simulink model "comfort"  (R2013b)
settings: Solver=ode45  StartTime=0.0  StopTime=0  RelTol=1e-3
undefined symbols (not defined in the file): CarnotCallbacks_PMV_PPD
settings Model: Creator=awohlfei  LastModifiedBy=drhf
settings DebuggingCC: SolverPrmCheckMsg=none  StateNameClashWarn=warning

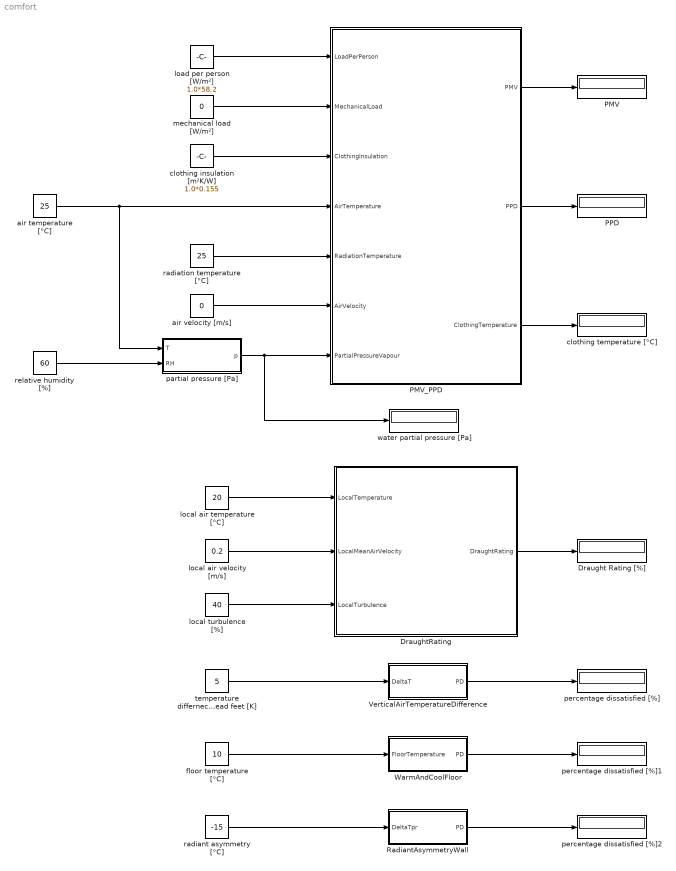
== system comfort ==
  Draught Rating [%] : Display
  DraughtRating : Subsystem  mask(Drauting Rate){}
      mask help: The block calculates the draut rate according to ISO 7730.
  PMV : Display
  PMV_PPD : Subsystem  LoadFcn=CarnotCallbacks_PMV_PPD('LoadFcn', gcb);  mask(PMV_PPD){DEBUGLEVEL=WARNINGLEVEL, MAXTOTALWARNINGS=inf, MAXCONSECUTIVEWARNINGS=inf, WRITETOFILE=0, FILENAME='messages.txt'}
      mask prompts: DEBUGLEVEL "Debug level"; MAXTOTALWARNINGS "maximum number of total warning"; MAXCONSECUTIVEWARNINGS "maximum number of consecutive warnings"; WRITETOFILE "write messages to file"; FILENAME "filename for messages"
      mask help: This block calculates from it's inputs the thermal comfort according to PMV (pedicted mean vote) and PPD (predicted percentage of dissatisfied).
      mask init:
      | %global debug level
      | [DEBUGLEVEL, MAXTOTALWARNINGS, MAXCONSECUTIVEWARNINGS, WRITETOFILE, FILENAME] = CarnotCallbacks_PMV_PPD('CheckDebugLevels', DEBUGLEVEL, MAXTOTALWARNINGS, MAXCONSECUTIVEWARNINGS, WRITETOFILE, FILENAME);
      mask TypeOptions DEBUGLEVEL: DEBUGLEVEL | INFOLEVEL | WARNINGLEVEL | ERRORLEVEL | FATALLEVEL | NOLEVEL
      mask Callback DEBUGLEVEL: CarnotCallbacks_PMV_PPD('MaskVisibilities');
  PPD : Display
  RadiantAsymmetryWall : Subsystem  mask(Radiant Asymmetry){SURROUNDING=wall}
      mask prompts: SURROUNDING "type of surrounding"
      mask help: The block calculates the percentage of dissatiesfied according to ISO 7730 in dempendence of the radiant asymmetry.
      mask TypeOptions SURROUNDING: wall | ceiling
  VerticalAirTemperatureDifference : Subsystem  mask(Vertical Temperature Difference){}
      mask help: This block calculates the percentage of dissatisfied depending on the temperature difference between head and feet according to ISO 7730.
  WarmAndCoolFloor : Subsystem  mask(Warm and Cool Floor){}
      mask help: The block calculates the percentage of dissatisfied in dependence of the floor temperature.
  air temperature [°C] : Constant  Value=25
  air velocity [m/s] : Constant  Value=0
  clothing insulation [m²K/W] : Constant  Value=1.0*0.155
  clothing temperature [°C] : Display
  floor temperature [°C] : Constant  Value=10
  load per person [W/m²] : Constant  Value=1.0*58.2
  local air temperature [°C] : Constant  Value=20
  local air velocity [m/s] : Constant  Value=0.2
  local turbulence [%] : Constant  Value=40
  mechanical load [W/m²] : Constant  Value=0
  partial pressure [Pa] : Subsystem
  percentage dissatisfied [%] : Display
  percentage dissatisfied [%]1 : Display
  percentage dissatisfied [%]2 : Display
  radiant asymmetry [°C] : Constant  Value=-15
  radiation temperature [°C] : Constant  Value=25
  relative humidity [%] : Constant  Value=60
  temperature differnece head feet [K] : Constant  Value=5
  water partial pressure [Pa] : Display
  wires:
  air temperature [°C]/1 -> partial pressure [Pa]/1(T), PMV_PPD/4(AirTemperature)
  relative humidity [%]/1 -> partial pressure [Pa]/2(RH)
  partial pressure [Pa]/1(p) -> water partial pressure [Pa]/1, PMV_PPD/7(PartialPressureVapour)
  load per person [W/m²]/1 -> PMV_PPD/1(LoadPerPerson)
  mechanical load [W/m²]/1 -> PMV_PPD/2(MechanicalLoad)
  clothing insulation [m²K/W]/1 -> PMV_PPD/3(ClothingInsulation)
  radiation temperature [°C]/1 -> PMV_PPD/5(RadiationTemperature)
  air velocity [m/s]/1 -> PMV_PPD/6(AirVelocity)
  PMV_PPD/1(PMV) -> PMV/1
  PMV_PPD/2(PPD) -> PPD/1
  PMV_PPD/3(ClothingTemperature) -> clothing temperature [°C]/1
  local air temperature [°C]/1 -> DraughtRating/1(LocalTemperature)
  local air velocity [m/s]/1 -> DraughtRating/2(LocalMeanAirVelocity)
  local turbulence [%]/1 -> DraughtRating/3(LocalTurbulence)
  DraughtRating/1(DraughtRating) -> Draught Rating [%]/1
  temperature differnece head feet [K]/1 -> VerticalAirTemperatureDifference/1(DeltaT)
  VerticalAirTemperatureDifference/1(PD) -> percentage dissatisfied [%]/1
  WarmAndCoolFloor/1(PD) -> percentage dissatisfied [%]1/1
  floor temperature [°C]/1 -> WarmAndCoolFloor/1(FloorTemperature)
  radiant asymmetry [°C]/1 -> RadiantAsymmetryWall/1(DeltaTpr)
  RadiantAsymmetryWall/1(PD) -> percentage dissatisfied [%]2/1

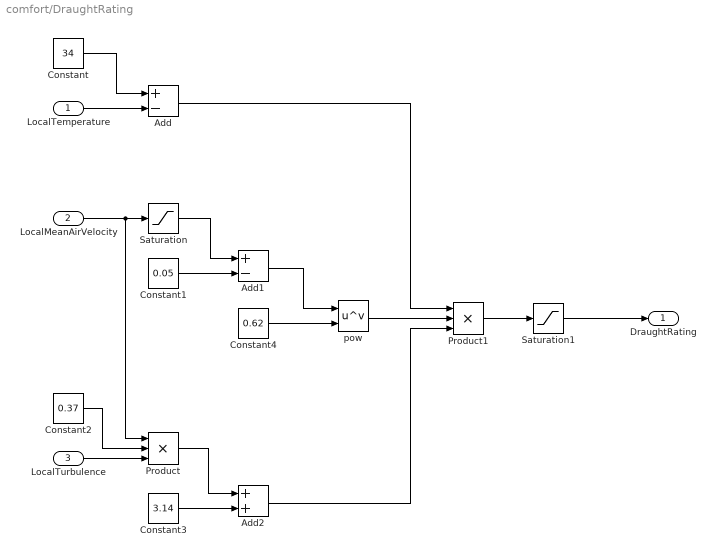
== system comfort/DraughtRating ==
  LocalTemperature : Inport
  LocalMeanAirVelocity : Inport  Port=2
  LocalTurbulence : Inport  Port=3
  Add : Sum  Inputs=+-
  Add1 : Sum  Inputs=+-
  Add2 : Sum
  Constant : Constant  Value=34
  Constant1 : Constant  Value=0.05
  Constant2 : Constant  Value=0.37
  Constant3 : Constant  Value=3.14
  Constant4 : Constant  Value=0.62
  Product : Product  Inputs=3
  Product1 : Product  Inputs=3
  Saturation : Saturate  UpperLimit=inf  LowerLimit=0.05
  Saturation1 : Saturate  UpperLimit=100  LowerLimit=0
  pow : Math  Operator=pow  SaturateOnIntegerOverflow=on
  DraughtRating : Outport
  wires:
  LocalMeanAirVelocity/1 -> Saturation/1, Product/1
  LocalTemperature/1 -> Add/2
  Constant/1 -> Add/1
  Saturation/1 -> Add1/1
  Constant1/1 -> Add1/2
  Add1/1 -> pow/1
  Constant4/1 -> pow/2
  Constant2/1 -> Product/2
  LocalTurbulence/1 -> Product/3
  Constant3/1 -> Add2/2
  Product/1 -> Add2/1
  Product1/1 -> Saturation1/1
  Saturation1/1 -> DraughtRating/1
  pow/1 -> Product1/2
  Add2/1 -> Product1/3
  Add/1 -> Product1/1

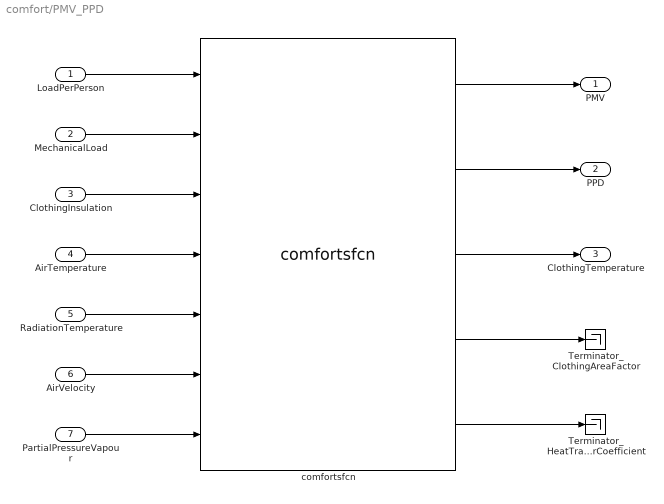
== system comfort/PMV_PPD ==
  LoadPerPerson : Inport
  MechanicalLoad : Inport  Port=2
  ClothingInsulation : Inport  Port=3
  AirTemperature : Inport  Port=4
  RadiationTemperature : Inport  Port=5
  AirVelocity : Inport  Port=6
  PartialPressureVapour : Inport  Port=7
  Terminator_ClothingAreaFactor : Terminator
  Terminator_HeatTransferCoefficient : Terminator
  comfortsfcn : S-Function  FunctionName=comfortsfcn  Parameters=DEBUGLEVEL-1, MAXTOTALWARNINGS, MAXCONSECUTIVEWARNINGS, WRITETOFILE, FILENAME  EnableBusSupport=off
  PMV : Outport
  PPD : Outport  Port=2
  ClothingTemperature : Outport  Port=3
  wires:
  PartialPressureVapour/1 -> comfortsfcn/7
  AirTemperature/1 -> comfortsfcn/4
  LoadPerPerson/1 -> comfortsfcn/1
  MechanicalLoad/1 -> comfortsfcn/2
  ClothingInsulation/1 -> comfortsfcn/3
  RadiationTemperature/1 -> comfortsfcn/5
  AirVelocity/1 -> comfortsfcn/6
  comfortsfcn/1 -> PMV/1
  comfortsfcn/2 -> PPD/1
  comfortsfcn/3 -> ClothingTemperature/1
  comfortsfcn/4 -> Terminator_ClothingAreaFactor/1
  comfortsfcn/5 -> Terminator_HeatTransferCoefficient/1

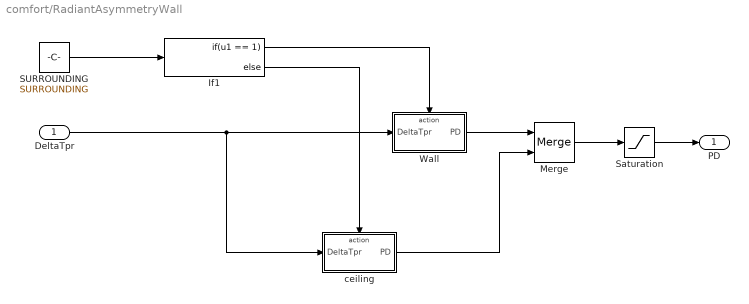
== system comfort/RadiantAsymmetryWall ==
  DeltaTpr : Inport
  If1 : If  IfExpression=u1 == 1
  Merge : Merge
  SURROUNDING : Constant  Value=SURROUNDING
  Saturation : Saturate  UpperLimit=100  LowerLimit=0
  Wall : Subsystem  TreatAsAtomicUnit=on
  ceiling : Subsystem  TreatAsAtomicUnit=on
  PD : Outport
  wires:
  Merge/1 -> Saturation/1
  SURROUNDING/1 -> If1/1
  If1/1 -> Wall/Action
  If1/2 -> ceiling/Action
  Wall/1(PD) -> Merge/1
  ceiling/1(PD) -> Merge/2
  DeltaTpr/1 -> ceiling/1(DeltaTpr), Wall/1(DeltaTpr)
  Saturation/1 -> PD/1

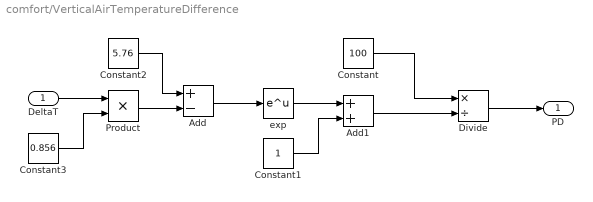
== system comfort/VerticalAirTemperatureDifference ==
  DeltaT : Inport
  Add : Sum  Inputs=+-
  Add1 : Sum
  Constant : Constant  Value=100
  Constant1 : Constant
  Constant2 : Constant  Value=5.76
  Constant3 : Constant  Value=0.856
  Divide : Product  Inputs=*/
  Product : Product
  exp : Math  SaturateOnIntegerOverflow=on
  PD : Outport
  wires:
  DeltaT/1 -> Product/1
  Constant3/1 -> Product/2
  Product/1 -> Add/2
  Constant2/1 -> Add/1
  Add/1 -> exp/1
  exp/1 -> Add1/1
  Constant1/1 -> Add1/2
  Constant/1 -> Divide/1
  Add1/1 -> Divide/2
  Divide/1 -> PD/1

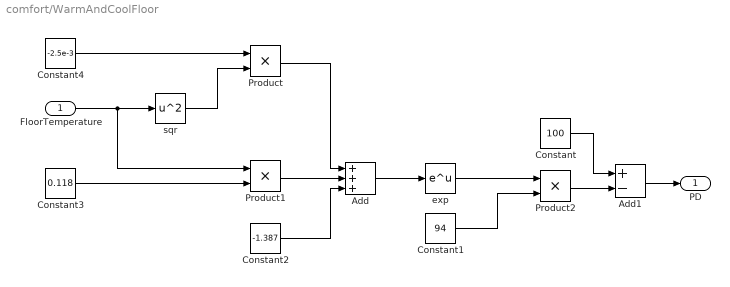
== system comfort/WarmAndCoolFloor ==
  FloorTemperature : Inport
  Add : Sum  Inputs=+++
  Add1 : Sum  Inputs=+-
  Constant : Constant  Value=100
  Constant1 : Constant  Value=94
  Constant2 : Constant  Value=-1.387
  Constant3 : Constant  Value=0.118
  Constant4 : Constant  Value=-2.5e-3
  Product : Product
  Product1 : Product
  Product2 : Product
  exp : Math  SaturateOnIntegerOverflow=on
  sqr : Math  Operator=square  SaturateOnIntegerOverflow=on
  PD : Outport
  wires:
  FloorTemperature/1 -> Product1/1, sqr/1
  Constant4/1 -> Product/1
  sqr/1 -> Product/2
  Constant3/1 -> Product1/2
  Product1/1 -> Add/2
  Product/1 -> Add/1
  Constant2/1 -> Add/3
  Add/1 -> exp/1
  Constant1/1 -> Product2/2
  exp/1 -> Product2/1
  Product2/1 -> Add1/2
  Constant/1 -> Add1/1
  Add1/1 -> PD/1

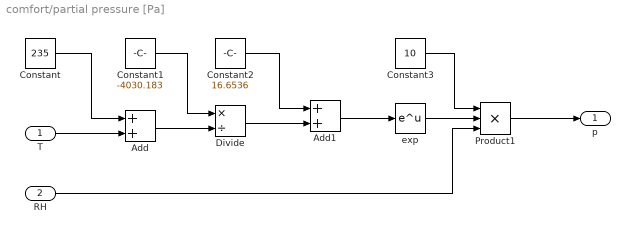
== system comfort/partial pressure [Pa] ==
  T : Inport
  RH : Inport  Port=2
  Add : Sum
  Add1 : Sum
  Constant : Constant  Value=235
  Constant1 : Constant  Value=-4030.183
  Constant2 : Constant  Value=16.6536
  Constant3 : Constant  Value=10
  Divide : Product  Inputs=*/
  Product1 : Product  Inputs=3
  exp : Math  SaturateOnIntegerOverflow=on
  p : Outport
  wires:
  Constant/1 -> Add/1
  T/1 -> Add/2
  Add/1 -> Divide/2
  Constant1/1 -> Divide/1
  Divide/1 -> Add1/2
  Constant2/1 -> Add1/1
  Add1/1 -> exp/1
  exp/1 -> Product1/2
  RH/1 -> Product1/3
  Constant3/1 -> Product1/1
  Product1/1 -> p/1

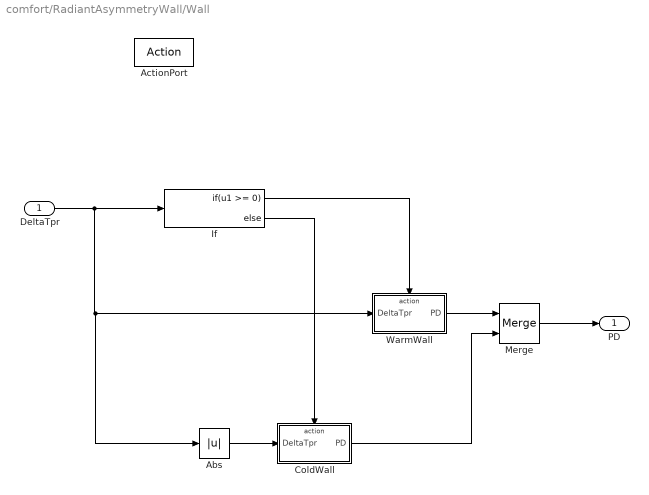
== system comfort/RadiantAsymmetryWall/Wall ==
  DeltaTpr : Inport
  ActionPort : ActionPort  ActionType=then
  Abs : Abs
  ColdWall : Subsystem  TreatAsAtomicUnit=on
  If : If  IfExpression=u1 >= 0
  Merge : Merge
  WarmWall : Subsystem  TreatAsAtomicUnit=on
  PD : Outport
  wires:
  DeltaTpr/1 -> Abs/1, WarmWall/1(DeltaTpr), If/1
  If/1 -> WarmWall/Action
  If/2 -> ColdWall/Action
  WarmWall/1(PD) -> Merge/1
  ColdWall/1(PD) -> Merge/2
  Merge/1 -> PD/1
  Abs/1 -> ColdWall/1(DeltaTpr)

== system comfort/RadiantAsymmetryWall/ceiling ==
  DeltaTpr : Inport
  ActionPort : ActionPort  ActionType=else
  Abs : Abs
  ColdCeiling : Subsystem  TreatAsAtomicUnit=on
  If : If  IfExpression=u1 >= 0
  Merge : Merge
  WarmCeiling : Subsystem  TreatAsAtomicUnit=on
  PD : Outport
  wires:
  Merge/1 -> PD/1
  ColdCeiling/1(PD) -> Merge/2
  WarmCeiling/1(PD) -> Merge/1
  If/2 -> ColdCeiling/Action
  If/1 -> WarmCeiling/Action
  DeltaTpr/1 -> If/1, WarmCeiling/1(DeltaTpr), Abs/1
  Abs/1 -> ColdCeiling/1(DeltaTpr)

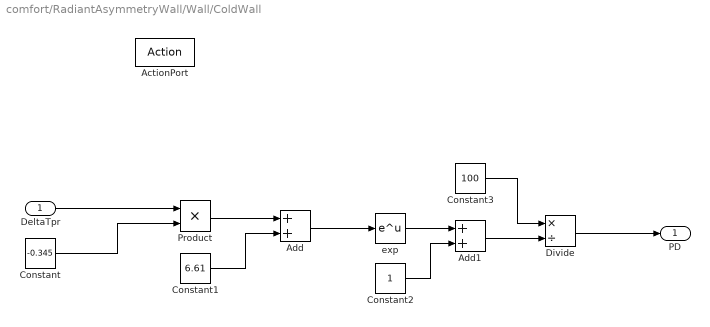
== system comfort/RadiantAsymmetryWall/Wall/ColdWall ==
  DeltaTpr : Inport
  ActionPort : ActionPort  ActionType=else
  Add : Sum
  Add1 : Sum
  Constant : Constant  Value=-0.345
  Constant1 : Constant  Value=6.61
  Constant2 : Constant
  Constant3 : Constant  Value=100
  Divide : Product  Inputs=*/
  Product : Product
  exp : Math  SaturateOnIntegerOverflow=on
  PD : Outport
  wires:
  Divide/1 -> PD/1
  Add1/1 -> Divide/2
  Constant3/1 -> Divide/1
  Constant2/1 -> Add1/2
  exp/1 -> Add1/1
  Add/1 -> exp/1
  Constant1/1 -> Add/2
  Product/1 -> Add/1
  Constant/1 -> Product/2
  DeltaTpr/1 -> Product/1

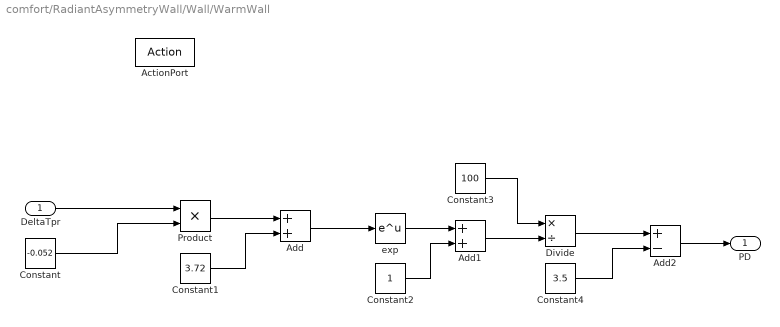
== system comfort/RadiantAsymmetryWall/Wall/WarmWall ==
  DeltaTpr : Inport
  ActionPort : ActionPort  ActionType=then
  Add : Sum
  Add1 : Sum
  Add2 : Sum  Inputs=+-
  Constant : Constant  Value=-0.052
  Constant1 : Constant  Value=3.72
  Constant2 : Constant
  Constant3 : Constant  Value=100
  Constant4 : Constant  Value=3.5
  Divide : Product  Inputs=*/
  Product : Product
  exp : Math  SaturateOnIntegerOverflow=on
  PD : Outport
  wires:
  DeltaTpr/1 -> Product/1
  Constant/1 -> Product/2
  Product/1 -> Add/1
  Constant1/1 -> Add/2
  Add/1 -> exp/1
  exp/1 -> Add1/1
  Constant2/1 -> Add1/2
  Constant3/1 -> Divide/1
  Add1/1 -> Divide/2
  Divide/1 -> Add2/1
  Constant4/1 -> Add2/2
  Add2/1 -> PD/1

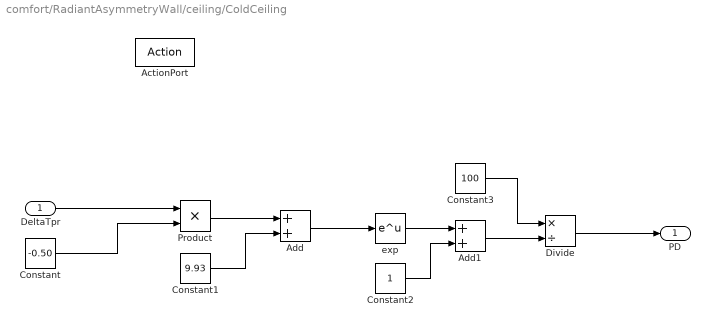
== system comfort/RadiantAsymmetryWall/ceiling/ColdCeiling ==
  DeltaTpr : Inport
  ActionPort : ActionPort  ActionType=else
  Add : Sum
  Add1 : Sum
  Constant : Constant  Value=-0.50
  Constant1 : Constant  Value=9.93
  Constant2 : Constant
  Constant3 : Constant  Value=100
  Divide : Product  Inputs=*/
  Product : Product
  exp : Math  SaturateOnIntegerOverflow=on
  PD : Outport
  wires:
  DeltaTpr/1 -> Product/1
  Constant/1 -> Product/2
  Product/1 -> Add/1
  Constant1/1 -> Add/2
  Add/1 -> exp/1
  exp/1 -> Add1/1
  Constant2/1 -> Add1/2
  Constant3/1 -> Divide/1
  Add1/1 -> Divide/2
  Divide/1 -> PD/1

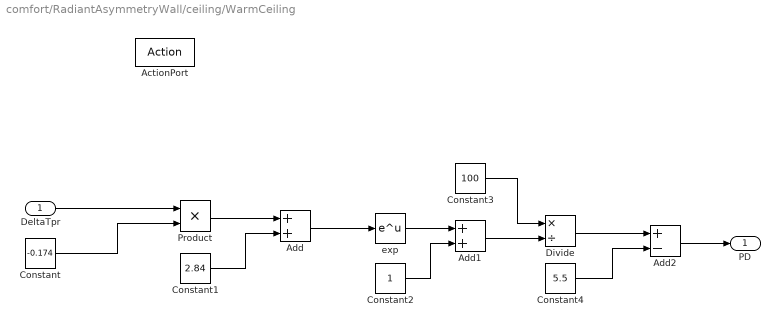
== system comfort/RadiantAsymmetryWall/ceiling/WarmCeiling ==
  DeltaTpr : Inport
  ActionPort : ActionPort  ActionType=then
  Add : Sum
  Add1 : Sum
  Add2 : Sum  Inputs=+-
  Constant : Constant  Value=-0.174
  Constant1 : Constant  Value=2.84
  Constant2 : Constant
  Constant3 : Constant  Value=100
  Constant4 : Constant  Value=5.5
  Divide : Product  Inputs=*/
  Product : Product
  exp : Math  SaturateOnIntegerOverflow=on
  PD : Outport
  wires:
  Add2/1 -> PD/1
  Constant4/1 -> Add2/2
  Divide/1 -> Add2/1
  Add1/1 -> Divide/2
  Constant3/1 -> Divide/1
  Constant2/1 -> Add1/2
  exp/1 -> Add1/1
  Add/1 -> exp/1
  Constant1/1 -> Add/2
  Product/1 -> Add/1
  Constant/1 -> Product/2
  DeltaTpr/1 -> Product/1
